simulink model "MIL4L3_SW6_V1_20220211"  (R2018b)
settings: Solver=FixedStepAuto  StartTime=0.0  StopTime=inf  FixedStep=0.001  RelTol=1e-3
PreLoadFcn:
  | A0_MILtest;
undefined symbols (not defined in the file or in its folder): Clb_ICADirect_LaneDisp_StateFive, Clb_ICADirect_LaneDisp_StateFour, Clb_ICADirect_LaneDisp_StateOne, Clb_ICADirect_LaneDisp_StateThree, Clb_ICADirect_LaneDisp_StateTwo, Clb_ICADirect_LaneDisp_StateZero, Clb_ICADirect_LaneDispSW, Clb_ICADirect_TrnLghtsCom_Switch, Clb_ICADirect_TrnLghtsCom_Value, Clb_ICADirect_TrnLghtsCrtl_Inhb, IMAP_Clb_ACU_Driver_Belt, IMAP_Clb_ACU_Driver_Belt_Over, IMAP_Clb_ACU_Passenger_Belt, IMAP_Clb_ACU_Passenger_Belt_Over, IMAP_Clb_ACU_RearLeft_Belt, IMAP_Clb_ACU_RearLeft_Belt_Over, IMAP_Clb_ACU_RearMiddle_Belt, IMAP_Clb_ACU_RearMiddle_Belt_Over, IMAP_Clb_ACU_RearRight_Belt, IMAP_Clb_ACU_RearRight_Belt_Over, IMAP_Clb_AEB_Switch, IMAP_Clb_AEB_Switch_Over, IMAP_Clb_ALC_TLC_Mode, IMAP_Clb_ALC_TLC_Mode_Over, IMAP_Clb_BCM_Battery_Voltage, IMAP_Clb_BCM_Battery_Voltage_Over, IMAP_Clb_BCM_BrakeLamp_State, IMAP_Clb_BCM_BrakeLamp_State_Over, IMAP_Clb_BCM_CHMSL_Status, IMAP_Clb_BCM_CHMSL_Status_Over, IMAP_Clb_BCM_Door_Lock_State, IMAP_Clb_BCM_Door_Lock_State_Over, IMAP_Clb_BCM_FrontWiper_State, IMAP_Clb_BCM_FrontWiper_State_Over, IMAP_Clb_BCM_FrontWiper_Switch, IMAP_Clb_BCM_FrontWiper_Switch_Over, IMAP_Clb_BCM_HazardLamp, IMAP_Clb_BCM_HazardLamp_Over, IMAP_Clb_BCM_HazardLamp_Switch, IMAP_Clb_BCM_HazardLamp_Switch_Over, IMAP_Clb_BCM_HighBeam_State, IMAP_Clb_BCM_HighBeam_State_Over, IMAP_Clb_BCM_Ignition_State, IMAP_Clb_BCM_Ignition_State_Over, IMAP_Clb_BCM_IHBC_Enabled, IMAP_Clb_BCM_IHBC_Enabled_Over, IMAP_Clb_BCM_Left_Light, IMAP_Clb_BCM_Left_Light_Over, IMAP_Clb_BCM_LeftTurn_Switch, IMAP_Clb_BCM_LeftTurn_Switch_Over, IMAP_Clb_BCM_LF_Door_State, IMAP_Clb_BCM_LF_Door_State_Over, IMAP_Clb_BCM_LowBeam_State, IMAP_Clb_BCM_LowBeam_State_Over, IMAP_Clb_BCM_LR_Door_State, IMAP_Clb_BCM_LR_Door_State_Over, IMAP_Clb_BCM_RF_Door_State, IMAP_Clb_BCM_RF_Door_State_Over, IMAP_Clb_BCM_Right_Light, IMAP_Clb_BCM_Right_Light_Over ... (+547)
libraries: CarMaker4SL x2153, simulink x292, dspstat3 x3, canmsglib x2, simulink_extras x1
(part 36 of 52)

== system MIL4L3_SW6_V1_20220211/CarMaker/VehicleControl/OMAP/OMAP1/Runnable_OMAP_10ms_sys/OMAP_Module/ESAS_Direct ==
  note: ESA为扭矩接口。那对应的角度接口的4个信号怎么发？
  Input_ESAS : Inport
  Input_FDMM : Inport  Port=2
  Bus Creator : BusCreator  Inputs=7
  Bus Creator14 : BusCreator  Inputs=8
  Bus Creator23 : BusCreator  Inputs=36
  Bus Creator5 : BusCreator  Inputs=13
  Bus Selector : BusSelector  OutputSignals=ESASve_g_EPS_Factor_Control_convert,ESASve_g_ESA_SWA_CMD_convert,ESASve_y_LKAActivation_convert,ESASve_y_ESA_State_convert,ESASve_y_ESATorqueReq_convert,ESASve_y_ESARequest_convert
  Bus Selector1 : BusSelector  OutputSignals=ESASve_y_ESA_FaultSt_convert
  Constant1 : Constant  Value=0  OutDataTypeStr=uint8
  Constant23 : Constant  Value=0  OutDataTypeStr=uint8
  Constant4 : Constant  Value=0  OutDataTypeStr=uint8
  Data Type Conversion{1..2,4,31} (4 alike) : DataTypeConversion  OutDataTypeStr=uint8
  Data Type Conversion29 : DataTypeConversion  OutDataTypeStr=single
  Data Type Conversion3 : DataTypeConversion  OutDataTypeStr=single
  Data Type Conversion30 : DataTypeConversion  OutDataTypeStr=single
  OMAPve_g_ACCTqReqNum : Constant  Value=-4000  OutDataTypeStr=single
  OMAPve_g_Deceleration_setpoint_deviceNum : Constant  Value=2.05  OutDataTypeStr=single
  OMAPve_g_PotACCTqReqNum : Constant  Value=-4000  OutDataTypeStr=single
  OMAPve_g_TminUp_or_downGearNum : Constant  Value=6.2  OutDataTypeStr=single
  OMAPve_y_ACC_DesiredHeadway_DisplayNum5 : Constant  Value=0  OutDataTypeStr=uint8
  OMAPve_y_ACC_DesiredHeadway_Icon_BasicNum5 : Constant  Value=0  OutDataTypeStr=uint8
  OMAPve_y_ACC_Desired_Set_SpeedNum5 : Constant  Value=0  OutDataTypeStr=uint8
  OMAPve_y_ACC_Engine_Start_RequestNum : Constant  Value=0  OutDataTypeStr=uint8
  OMAPve_y_ACC_HMI_TgtDisp_FlagNum5 : Constant  Value=0  OutDataTypeStr=uint8
  OMAPve_y_ACC_Pop_Up_MessageNum5 : Constant  Value=0  OutDataTypeStr=uint8
  OMAPve_y_ACC_Set_Speed_DisplayNum5 : Constant  Value=0  OutDataTypeStr=uint8
  OMAPve_y_ACC_Vehicle_Icon_DisplayNum5 : Constant  Value=0  OutDataTypeStr=uint8
  OMAPve_y_ADAS_ACCRequestEPBNum : Constant  Value=0  OutDataTypeStr=uint8
  OMAPve_y_ADAS_ELKStsNum1 : Constant  Value=0  OutDataTypeStr=uint8
  OMAPve_y_ADAS_ESCDriveOffNum : Constant  Value=0  OutDataTypeStr=uint8
  OMAPve_y_ADAS_ESCHoldReqNum : Constant  Value=0  OutDataTypeStr=uint8
  OMAPve_y_ADAS_HWAActionSts : Constant  Value=0  OutDataTypeStr=uint8
  OMAPve_y_ADAS_HWAMode : Constant  Value=0  OutDataTypeStr=uint8
  OMAPve_y_ADAS_HWATurnOnIndicator : Constant  Value=0  OutDataTypeStr=uint8
  OMAPve_y_ADAS_ISLCDriverRemind1 : Constant  Value=0  OutDataTypeStr=uint8
  OMAPve_y_ADAS_ISLCState1 : Constant  Value=0  OutDataTypeStr=uint8
  OMAPve_y_ADAS_JAFaultSt_2 : Constant  Value=0  OutDataTypeStr=uint8
  OMAPve_y_ADAS_LightControlValid : Constant  Value=0  OutDataTypeStr=uint8
  OMAPve_y_ADAS_TurnLightsCommand1 : Constant  Value=0  OutDataTypeStr=uint8
  OMAPve_y_AEB_Alert_ReqNum3 : Constant  Value=0  OutDataTypeStr=uint8
  OMAPve_y_AEB_Braking_progressNum : Constant  Value=0  OutDataTypeStr=uint8
  OMAPve_y_AEB_Fault_StatusNum3 : Constant  Value=0  OutDataTypeStr=uint8
  OMAPve_y_AEB_StatusNum : Constant  Value=0  OutDataTypeStr=uint8
  OMAPve_y_AEB_Switch_StatusNum3 : Constant  Value=0  OutDataTypeStr=uint8
  OMAPve_y_AEB_tipsNum3 : Constant  Value=0  OutDataTypeStr=uint8
  OMAPve_y_Decel_RequestNum : Constant  Value=0  OutDataTypeStr=uint8
  OMAPve_y_FCW_StatusNum : Constant  Value=10  OutDataTypeStr=uint8
  OMAPve_y_Function_Acc_statusNum : Constant  Value=3  OutDataTypeStr=uint8
  OMAPve_y_HMI_Popup_StatusNum3 : Constant  Value=0  OutDataTypeStr=uint8
  OMAPve_y_Hands_off_warningNum3 : Constant  Value=0  OutDataTypeStr=uint8
  OMAPve_y_Haptic_AlarmNum : Constant  Value=0  OutDataTypeStr=uint8
  OMAPve_y_ICA_HMI_Txt_DispNum5 : Constant  Value=0  OutDataTypeStr=uint8
  OMAPve_y_LDW_FlagNum4 : Constant  Value=0  OutDataTypeStr=uint8
  OMAPve_y_LDW_Status_DisplayNum4 : Constant  Value=0  OutDataTypeStr=uint8
  OMAPve_y_LKA_Mode_from_CameraNum4 : Constant  Value=0  OutDataTypeStr=uint8
  OMAPve_y_LKA_Status_DisplayNum3 : Constant  Value=0  OutDataTypeStr=uint8
  OMAPve_y_LKA_Switch_StateNum4 : Constant  Value=0  OutDataTypeStr=uint8
  OMAPve_y_LKA_action_indicationNum3 : Constant  Value=0  OutDataTypeStr=uint8
  OMAPve_y_MDD_Decelerationcontrol_requestNum : Constant  Value=0  OutDataTypeStr=uint8
  OMAPve_y_MDD_deceleration_typeNum : Constant  Value=0  OutDataTypeStr=uint8
  OMAPve_y_Powertrain_torquewheel_requestNum : Constant  Value=0  OutDataTypeStr=uint8
  OMAPve_y_Prefill_requestNum : Constant  Value=0  OutDataTypeStr=uint8
  OMAPve_y_RVVACC_Vehiclespeed_request_typeNum5 : Constant  Value=0  OutDataTypeStr=uint8
  OMAPve_y_State_of_the_functionFARC_detNum : Constant  Value=0  OutDataTypeStr=uint8
  OMAPve_y_TARGET_POSITIONNum5 : Constant  Value=6  OutDataTypeStr=uint8
  OMAPve_y_TJA_status_iconNum5 : Constant  Value=0  OutDataTypeStr=uint8
  OMAPve_y_TSR_Vision_Only_Sign_TypeNum5 : Constant  Value=0  OutDataTypeStr=uint8
  OMAPve_y_Vehicle_Lane_DisplayNum4 : Constant  Value=0  OutDataTypeStr=uint8
  OMAPve_y_stAcvTqWhlPTPotReqNum : Constant  Value=0  OutDataTypeStr=uint8
  Terminator1 : Terminator
  ESA_EMS : Outport
  ESA_ESC : Outport  Port=2
  ESA_EPS : Outport  Port=3
  ESA_IC : Outport  Port=4
  wires:
  Bus Creator23/1 -> ESA_IC/1  "ESA_IC"
  Bus Creator14/1 -> ESA_EPS/1  "ESA_EPS"
  OMAPve_y_AEB_Fault_StatusNum3/1 -> Bus Creator23/17  "OMAPve_y_AEB_Fault_Status_2"
  OMAPve_y_ACC_Vehicle_Icon_DisplayNum5/1 -> Bus Creator23/13  "OMAPve_y_ACC_Vehicle_Icon_Display_2"
  OMAPve_y_TSR_Vision_Only_Sign_TypeNum5/1 -> Bus Creator23/8  "OMAPve_y_TSR_Vision_Only_Sign_Type_2"
  OMAPve_y_AEB_Alert_ReqNum3/1 -> Bus Creator23/16  "OMAPve_y_AEB_Alert_Req_2"
  OMAPve_y_TJA_status_iconNum5/1 -> Bus Creator23/36  "OMAPve_y_TJA_status_icon_2"
  OMAPve_y_TARGET_POSITIONNum5/1 -> Bus Creator23/22  "OMAPve_y_TARGET_POSITION_2"
  OMAPve_y_AEB_Switch_StatusNum3/1 -> Bus Creator23/18  "OMAPve_y_AEB_Switch_Status_2"
  OMAPve_y_AEB_tipsNum3/1 -> Bus Creator23/19  "OMAPve_y_AEB_tips_2"
  OMAPve_y_ICA_HMI_Txt_DispNum5/1 -> Bus Creator23/35  "OMAPve_y_ICA_HMI_Txt_Disp_2"
  OMAPve_y_ACC_Desired_Set_SpeedNum5/1 -> Bus Creator23/11  "OMAPve_y_ACC_Desired_Set_Speed_2"
  OMAPve_y_ACC_DesiredHeadway_DisplayNum5/1 -> Bus Creator23/9  "OMAPve_y_ACC_DesiredHeadway_Display_2"
  OMAPve_y_LKA_Switch_StateNum4/1 -> Bus Creator23/32  "OMAPve_y_LKA_Switch_State_2"
  OMAPve_y_LKA_Status_DisplayNum3/1 -> Bus Creator23/31  "OMAPve_y_LKA_Status_Display_2"
  OMAPve_y_LDW_Status_DisplayNum4/1 -> Bus Creator23/29  "OMAPve_y_LDW_Status_Display_2"
  OMAPve_y_ACC_Pop_Up_MessageNum5/1 -> Bus Creator23/15  "OMAPve_y_ACC_Pop_Up_Message_2"
  OMAPve_y_ACC_Set_Speed_DisplayNum5/1 -> Bus Creator23/12  "OMAPve_y_ACC_Set_Speed_Display_2"
  Data Type Conversion30/1 -> Bus Creator14/4  "OMAPve_g_Column_angle_setpoint3F2_2"
  OMAPve_y_HMI_Popup_StatusNum3/1 -> Bus Creator23/26  "OMAPve_y_HMI_Popup_Status_2"
  OMAPve_y_Vehicle_Lane_DisplayNum4/1 -> Bus Creator23/27  "OMAPve_y_Vehicle_Lane_Display_2"
  OMAPve_y_ACC_HMI_TgtDisp_FlagNum5/1 -> Bus Creator23/21  "OMAPve_y_ACC_HMI_TgtDisp_Flag_2"
  Data Type Conversion29/1 -> Bus Creator14/3  "OMAPve_g_Coefficient_toregulate_EPS_2"
  OMAPve_y_Hands_off_warningNum3/1 -> Bus Creator23/25  "OMAPve_y_Hands_off_warning_2"
  OMAPve_y_LKA_action_indicationNum3/1 -> Bus Creator23/33  "OMAPve_y_LKA_action_indication_2"
  OMAPve_y_LKA_Mode_from_CameraNum4/1 -> Bus Creator23/30  "OMAPve_y_LKA_Mode_from_Camera_2"
  Constant1/1 -> Bus Creator14/2  "OMAPve_y_General_state_of_LKA_function3F2_2"
  OMAPve_y_RVVACC_Vehiclespeed_request_typeNum5/1 -> Bus Creator23/14  "OMAPve_y_RVVACC_Vehiclespeed_request_type_2"
  Data Type Conversion31/1 -> Bus Creator14/5  "OMAPve_y_Permit_to_know_if_LKA_or_LPA3F2_2"
  OMAPve_y_LDW_FlagNum4/1 -> Bus Creator23/28  "OMAPve_y_LDW_Flag_2"
  Constant23/1 -> Bus Creator14/1  "OMAPve_y_Power_steering_power_cut3F2_2"
  OMAPve_y_ACC_DesiredHeadway_Icon_BasicNum5/1 -> Bus Creator23/10  "OMAPve_y_ACC_DesiredHeadway_Icon_Basic_2"
  OMAPve_y_State_of_the_functionFARC_detNum/1 -> Bus Creator5/2  "OMAPve_y_State_of_the_functionFARC_det_1"
  OMAPve_y_Haptic_AlarmNum/1 -> Bus Creator5/5  "OMAPve_y_Haptic_Alarm_1"
  OMAPve_y_FCW_StatusNum/1 -> Bus Creator5/1  "OMAPve_y_FCW_Status_1"
  OMAPve_y_MDD_deceleration_typeNum/1 -> Bus Creator5/10  "OMAPve_y_MDD_deceleration_type_1"
  Bus Creator5/1 -> ESA_ESC/1  "ESA_ESC"
  OMAPve_y_MDD_Decelerationcontrol_requestNum/1 -> Bus Creator5/9  "OMAPve_y_MDD_Decelerationcontrol_request_1"
  OMAPve_y_AEB_Braking_progressNum/1 -> Bus Creator5/12  "OMAPve_y_AEB_Braking_progress_1"
  OMAPve_y_AEB_StatusNum/1 -> Bus Creator5/3  "OMAPve_y_AEB_Status_1"
  OMAPve_g_Deceleration_setpoint_deviceNum/1 -> Bus Creator5/8  "OMAPve_g_Deceleration_setpoint_device_1"
  OMAPve_g_ACCTqReqNum/1 -> Bus Creator/3  "OMAPve_g_ACCTqReq_1"
  Bus Creator/1 -> ESA_EMS/1  "ESA_EMS"
  OMAPve_g_PotACCTqReqNum/1 -> Bus Creator/2  "OMAPve_g_PotACCTqReq_1"
  OMAPve_y_ACC_Engine_Start_RequestNum/1 -> Bus Creator/1  "OMAPve_y_ACC_Engine_Start_Request_1"
  OMAPve_y_stAcvTqWhlPTPotReqNum/1 -> Bus Creator/6  "OMAPve_y_stAcvTqWhlPTPotReq_1"
  OMAPve_y_Decel_RequestNum/1 -> Bus Creator5/11  "OMAPve_y_Decel_Request_1"
  OMAPve_y_Function_Acc_statusNum/1 -> Bus Creator/7  "OMAPve_y_Function_Acc_status_1"
  OMAPve_g_TminUp_or_downGearNum/1 -> Bus Creator/5  "OMAPve_g_TminUp_or_downGear_1"
  OMAPve_y_Prefill_requestNum/1 -> Bus Creator5/4  "OMAPve_y_Prefill_request_1"
  OMAPve_y_Powertrain_torquewheel_requestNum/1 -> Bus Creator/4  "OMAPve_y_Powertrain_torquewheel_request_1"
  Input_FDMM/1 -> Terminator1/1
  OMAPve_y_ADAS_ELKStsNum1/1 -> Bus Creator23/34  "OMAPve_y_ADAS_ELKSts_2"
  OMAPve_y_ADAS_ESCHoldReqNum/1 -> Bus Creator5/7  "OMAPve_y_ADAS_ESCHoldReq"
  OMAPve_y_ADAS_ESCDriveOffNum/1 -> Bus Creator5/6  "OMAPve_y_ADAS_ESCDriveOff"
  OMAPve_y_ADAS_ACCRequestEPBNum/1 -> Bus Creator5/13  "OMAPve_y_ADAS_ACCRequestEPB"
  OMAPve_y_ADAS_JAFaultSt_2/1 -> Bus Creator23/20  "OMAPve_y_ADAS_JAFaultSt_2"
  OMAPve_y_ADAS_ISLCState1/1 -> Bus Creator23/23  "OMAPve_y_ADAS_ISLCState_2"
  OMAPve_y_ADAS_ISLCDriverRemind1/1 -> Bus Creator23/24  "OMAPve_y_ADAS_ISLCDriverRemind_2"
  OMAPve_y_ADAS_HWAActionSts/1 -> Bus Creator23/4  "OMAPve_y_ADAS_HWAActionSts_2"
  OMAPve_y_ADAS_HWAMode/1 -> Bus Creator23/7  "OMAPve_y_ADAS_HWAMode_2"
  OMAPve_y_ADAS_TurnLightsCommand1/1 -> Bus Creator23/5  "OMAPve_y_ADAS_TurnLightsCommand_2"
  OMAPve_y_ADAS_HWATurnOnIndicator/1 -> Bus Creator23/3  "OMAPve_y_ADAS_HWATurnOnIndicator_2"
  OMAPve_y_ADAS_LightControlValid/1 -> Bus Creator23/6  "OMAPve_y_ADAS_LightControlValid_2"
  Input_ESAS/1 -> Bus Selector1/1, Bus Selector/1
  Bus Selector/1 -> Data Type Conversion29/1  "<ESASve_g_EPS_Factor_Control_convert>"
  Bus Selector/2 -> Data Type Conversion30/1  "<ESASve_g_ESA_SWA_CMD_convert>"
  Bus Selector/3 -> Data Type Conversion31/1  "<ESASve_y_LKAActivation_convert>"
  Bus Selector/4 -> Data Type Conversion1/1  "<ESASve_y_ESA_State_convert>"
  Data Type Conversion1/1 -> Bus Creator14/6  "OMAPve_y_ADAS_ESAState_2"
  Bus Selector/6 -> Data Type Conversion2/1  "<ESASve_y_ESARequest_convert>"
  Data Type Conversion2/1 -> Bus Creator14/8  "OMAPve_y_ADAS_ESARequest_2"
  Bus Selector/5 -> Data Type Conversion3/1  "<ESASve_y_ESATorqueReq_convert>"
  Data Type Conversion3/1 -> Bus Creator14/7  "OMAPve_g_ADAS_ESATorqueReq_2"
  Data Type Conversion4/1 -> Bus Creator23/2  "OMAPve_y_ADAS_ESAFaultSt_2"
  Bus Selector1/1 -> Data Type Conversion4/1  "<ESASve_y_ESA_FaultSt_convert>"
  Constant4/1 -> Bus Creator23/1  "OMAPve_y_ADAS_ELKPopupMessage_2"

== system MIL4L3_SW6_V1_20220211/CarMaker/VehicleControl/OMAP/OMAP1/Runnable_OMAP_10ms_sys/OMAP_Module/ICA_Direct_G59 ==
  note: 配OMAP_G59
  note: 修改内容：G59 ET0车上与EPS的握手信号
      | 24 :增加转向灯命令信号，并为此信号增加两个标定量
      | 25:首次适配G59HMI，将车道线显示、文字显示、图标显示、声音提示均进行了适配修改，同时新增变道功能相关输出信号OMAPve_y_ADAS_HWATurnOnIndicator_2（请驾驶员拨转向杆确认变道）、OMAPve_y_ADAS_HWAActionSts_2（显示正在往左或是往右变道画面）、OMAPve_y_ADAS_LightControlValid_2（ADAS控转向灯有效性）、OMAPve_y_ADAS_TurnLightsCommand_2（ADAS控转向灯信号）、OMAPve_y_ADAS_HWAMode_2（多车道模式图标信号）。
      | 参考文档：OMAP接口文档3.6、HMI显示需求1.4、信号矩阵V2.1
      | 匹配模型：OMAP_ver032
      | 26:LKA activation控车与否都输出0
      | 27：取消降级达到恢复超时后橙色闪烁的设计，接入ICA模式开关信号、变道打转向灯信号，为HWATurnOnIndicator接入内容
      | 28：驾驶员立即接管触发条件新增车辆非静止
      | 29：经与G35商议一致，取消进入降级时的警示音（handsoffwarning）；把运算中的TH_MODE换为TH_STATE；增加标定量Clb_ICADirect_TrnLghtsCrtl_Inhb指示是否禁止控转向灯
      | 30:当ACC切ICA时，亮黄灯；从头开始开启ICA时，保持亮灰灯
      | 31：把上次改过的ICA icon这一块做了标定量，方便以后调试
      | 32:根据实车测试结果，实施ICA_ICON的更改，优化ACC切ICA时的HMI连续性; 根据对G35等竞品调研，增加扭矩系数变化率相关标定量
      | 33：修改车道线显示模块，显示方式设置两种，简单的只显示双灰双蓝，或者可显示单侧车道线，调试后确定一种；增加显示数值标定量。
      | 34：适配ICAB SW6的输出接口变动，删除部分无用信号，新增变道失败标志位
  Input_ICA : Inport
  Input_FDMM : Inport  Port=2
  Input_IMAP : Inport  Port=3
  ACC_to_ICA : Inport  Port=4
  Bus Creator : BusCreator  Inputs=2
  Bus Creator15 : BusCreator  Inputs=8
  Bus Creator24 : BusCreator  Inputs=36
  Bus Selector : BusSelector  OutputSignals=OMAPve_y_General_state_of_LKA_function3F2_2,OMAPve_g_Coefficient_toregulate_EPS_2,ICABve_g_SteerAngleCmd_convert,OMAPve_y_Permit_to_know_if_LKA_or_LPA3F2_2,ICABve_d_LKATorqueReq_convert,ICABve_g_LKATorqueReq_Value_convert
  Bus Selector1 : BusSelector  OutputSignals=OMAPve_y_ADAS_HWATurnOnIndicator_2,OMAPve_y_ADAS_HWAActionSts_2,OMAPve_y_ADAS_TurnLightsCommand_2,OMAPve_y_ADAS_LightControlValid_2,OMAPve_y_ADAS_HWAMode_2,OMAPve_y_TSR_Vision_Only_Sign_Type_2,OMAPve_y_ISA_Value_2,OMAPve_y_Hands_off_warning_2,OMAPve_y_Vehicle_Lane_Display_2,OMAPve_y_ICA_HMI_Txt_Disp_2,OMAPve_y_TJA_status_icon_2
  Bus Selector2 : BusSelector  OutputSignals=OMAPve_y_ACC_DesiredHeadway_Display_2,OMAPve_y_ACC_DesiredHeadway_Icon_Basic_2,OMAPve_y_ACC_Desired_Set_Speed_2,OMAPve_y_ACC_Set_Speed_Display_2,OMAPve_y_ACC_Vehicle_Icon_Display_2,OMAPve_y_RVVACC_Vehiclespeed_request_type_2,ACCSve_d_ACCMessagePrompt_convert,OMAPve_y_ACC_HMI_TgtDisp_Flag_2,OMAPve_y_TARGET_POSITION_2,ACCSve_d_ACC_ISLCState_convert,ACCSve_d_ACC_ISLCDriverRemind_convert
  Constant{,2..4} (4 alike) : Constant  Value=0  OutDataTypeStr=uint8
  Constant1 : Constant  Value=0  OutDataTypeStr=single
  Constant27 : Constant  Value=34  OutDataTypeStr=uint16
  Data Type Conversion1 : DataTypeConversion  OutDataTypeStr=single
  Data Type Conversion{3..5,7..20,22..25,28,46..47} (24 alike) : DataTypeConversion  OutDataTypeStr=uint8
  Data Type Conversion2 : DataTypeConversion  OutDataTypeStr=single
  Data Type Conversion21 : DataTypeConversion  OutDataTypeStr=single
  ICA_Define : Subsystem
  OMAPve_y_ADAS_ELKStsNum1 : Constant  Value=0  OutDataTypeStr=uint8
  OMAPve_y_ADAS_JAFaultSt_2 : Constant  Value=0  OutDataTypeStr=uint8
  OMAPve_y_AEB_Alert_ReqNum4 : Constant  Value=0  OutDataTypeStr=uint8
  OMAPve_y_AEB_Fault_StatusNum4 : Constant  Value=0  OutDataTypeStr=uint8
  OMAPve_y_AEB_Switch_StatusNum4 : Constant  Value=0  OutDataTypeStr=uint8
  OMAPve_y_AEB_tipsNum4 : Constant  Value=0  OutDataTypeStr=uint8
  OMAPve_y_HMI_Popup_StatusNum4 : Constant  Value=0  OutDataTypeStr=uint8
  OMAPve_y_LDW_FlagNum5 : Constant  Value=0  OutDataTypeStr=uint8
  OMAPve_y_LDW_Status_DisplayNum5 : Constant  Value=0  OutDataTypeStr=uint8
  OMAPve_y_LKA_Mode_from_CameraNum5 : Constant  Value=0  OutDataTypeStr=uint8
  OMAPve_y_LKA_Status_DisplayNum4 : Constant  Value=0  OutDataTypeStr=uint8
  OMAPve_y_LKA_Switch_StateNum5 : Constant  Value=0  OutDataTypeStr=uint8
  OMAPve_y_LKA_action_indicationNum4 : Constant  Value=0  OutDataTypeStr=uint8
  OMAPve_y_Power_steering_power_cut3F2Num2 : Constant  Value=0  OutDataTypeStr=uint8
  Terminator : Terminator
  Terminator1 : Terminator
  Terminator2 : Terminator
  ICA_EPS : Outport
  ICA_IC : Outport  Port=2
  ICA_Input : Outport  Port=3
  wires:
  OMAPve_y_AEB_Alert_ReqNum4/1 -> Bus Creator24/16  "OMAPve_y_AEB_Alert_Req_2"
  Data Type Conversion16/1 -> Bus Creator24/14  "OMAPve_y_RVVACC_Vehiclespeed_request_type_2"
  Bus Selector1/8 -> Data Type Conversion7/1  "<OMAPve_y_Hands_off_warning_2>"
  Data Type Conversion12/1 -> Bus Creator24/10  "OMAPve_y_ACC_DesiredHeadway_Icon_Basic_2"
  Bus Selector1/7 -> ?  "<OMAPve_y_ISA_Value_2>"
  Data Type Conversion14/1 -> Bus Creator24/12  "OMAPve_y_ACC_Set_Speed_Display_2"
  OMAPve_y_LDW_FlagNum5/1 -> Bus Creator24/28  "OMAPve_y_LDW_Flag_2"
  Bus Creator24/1 -> ICA_IC/1  "ICA_IC"
  OMAPve_y_AEB_tipsNum4/1 -> Bus Creator24/19  "OMAPve_y_AEB_tips_2"
  Bus Selector1/11 -> Data Type Conversion9/1  "<OMAPve_y_TJA_status_icon_2>"
  Data Type Conversion13/1 -> Bus Creator24/11  "OMAPve_y_ACC_Desired_Set_Speed_2"
  OMAPve_y_LKA_Status_DisplayNum4/1 -> Bus Creator24/31  "OMAPve_y_LKA_Status_Display_2"
  Data Type Conversion18/1 -> Bus Creator24/21  "OMAPve_y_ACC_HMI_TgtDisp_Flag_2"
  Data Type Conversion17/1 -> Bus Creator24/15  "OMAPve_y_ACC_Pop_Up_Message_2"
  OMAPve_y_LKA_Switch_StateNum5/1 -> Bus Creator24/32  "OMAPve_y_LKA_Switch_State_2"
  Data Type Conversion15/1 -> Bus Creator24/13  "OMAPve_y_ACC_Vehicle_Icon_Display_2"
  Bus Selector1/10 -> Data Type Conversion10/1  "<OMAPve_y_ICA_HMI_Txt_Disp_2>"
  OMAPve_y_LKA_Mode_from_CameraNum5/1 -> Bus Creator24/30  "OMAPve_y_LKA_Mode_from_Camera_2"
  OMAPve_y_LDW_Status_DisplayNum5/1 -> Bus Creator24/29  "OMAPve_y_LDW_Status_Display_2"
  OMAPve_y_AEB_Fault_StatusNum4/1 -> Bus Creator24/17  "OMAPve_y_AEB_Fault_Status_2"
  Bus Selector1/6 -> Data Type Conversion4/1  "<OMAPve_y_TSR_Vision_Only_Sign_Type_2>"
  OMAPve_y_HMI_Popup_StatusNum4/1 -> Bus Creator24/26  "OMAPve_y_HMI_Popup_Status_2"
  Bus Creator15/1 -> ICA_EPS/1  "ICA_EPS"
  Data Type Conversion11/1 -> Bus Creator24/9  "OMAPve_y_ACC_DesiredHeadway_Display_2"
  Data Type Conversion19/1 -> Bus Creator24/22  "OMAPve_y_TARGET_POSITION_2"
  OMAPve_y_AEB_Switch_StatusNum4/1 -> Bus Creator24/18  "OMAPve_y_AEB_Switch_Status_2"
  OMAPve_y_LKA_action_indicationNum4/1 -> Bus Creator24/33  "OMAPve_y_LKA_action_indication_2"
  Bus Selector1/9 -> Data Type Conversion8/1  "<OMAPve_y_Vehicle_Lane_Display_2>"
  Input_ICA/1 -> ICA_Define/1(In1)
  Input_IMAP/1 -> ICA_Define/3(In2)
  Input_FDMM/1 -> ICA_Define/2(In3)
  ACC_to_ICA/1 -> Bus Selector2/1, ICA_Define/4(In4)
  ICA_Define/2(Out2) -> Bus Creator/2, Bus Selector1/1  "HMI"
  Bus Creator/1 -> ICA_Input/1
  Data Type Conversion4/1 -> Bus Creator24/8  "OMAPve_y_TSR_Vision_Only_Sign_Type_2"
  Data Type Conversion7/1 -> Bus Creator24/25  "OMAPve_y_Hands_off_warning_2"
  Data Type Conversion8/1 -> Bus Creator24/27  "OMAPve_y_Vehicle_Lane_Display_2"
  Data Type Conversion9/1 -> Bus Creator24/36  "OMAPve_y_TJA_status_icon_2"
  Data Type Conversion10/1 -> Bus Creator24/35  "OMAPve_y_ICA_HMI_Txt_Disp_2"
  Bus Selector2/1 -> Data Type Conversion11/1  "<OMAPve_y_ACC_DesiredHeadway_Display_2>"
  Bus Selector2/2 -> Data Type Conversion12/1  "<OMAPve_y_ACC_DesiredHeadway_Icon_Basic_2>"
  Bus Selector2/3 -> Data Type Conversion13/1  "<OMAPve_y_ACC_Desired_Set_Speed_2>"
  Bus Selector2/4 -> Data Type Conversion14/1  "<OMAPve_y_ACC_Set_Speed_Display_2>"
  Bus Selector2/5 -> Data Type Conversion15/1  "<OMAPve_y_ACC_Vehicle_Icon_Display_2>"
  Bus Selector2/6 -> Data Type Conversion16/1  "<OMAPve_y_RVVACC_Vehiclespeed_request_type_2>"
  Bus Selector2/7 -> Data Type Conversion17/1  "<ACCSve_d_ACCMessagePrompt_convert>"
  Bus Selector2/8 -> Data Type Conversion18/1  "<OMAPve_y_ACC_HMI_TgtDisp_Flag_2>"
  Bus Selector2/9 -> Data Type Conversion19/1  "<OMAPve_y_TARGET_POSITION_2>"
  OMAPve_y_ADAS_ELKStsNum1/1 -> Bus Creator24/34  "OMAPve_y_ADAS_ELKSts_2"
  Data Type Conversion3/1 -> Bus Creator15/5  "OMAPve_y_Permit_to_know_if_LKA_or_LPA3F2_2"
  Bus Selector/5 -> Data Type Conversion20/1  "<ICABve_d_LKATorqueReq_convert>"
  Bus Selector/1 -> Data Type Conversion28/1  "<OMAPve_y_General_state_of_LKA_function3F2_2>"
  Bus Selector/4 -> Data Type Conversion3/1  "<OMAPve_y_Permit_to_know_if_LKA_or_LPA3F2_2>"
  Bus Selector/6 -> Data Type Conversion21/1  "<ICABve_g_LKATorqueReq_Value_convert>"
  Data Type Conversion20/1 -> Terminator/1  "OMAPve_y_DAS4_Status_LKATorqueReq"
  Bus Selector/2 -> Data Type Conversion1/1  "<OMAPve_g_Coefficient_toregulate_EPS_2>"
  OMAPve_y_Power_steering_power_cut3F2Num2/1 -> Bus Creator15/1  "OMAPve_y_Power_steering_power_cut3F2_2"
  Data Type Conversion1/1 -> Bus Creator15/3  "OMAPve_g_Coefficient_toregulate_EPS_2"
  Data Type Conversion28/1 -> Bus Creator15/2  "OMAPve_y_General_state_of_LKA_function3F2_2"
  Data Type Conversion21/1 -> Terminator1/1  "OMAPve_g_DAS4_Status_LKATorqueReq_Value"
  ICA_Define/1(Out1) -> Bus Selector/1, Bus Creator/1  "actuator"
  Bus Selector/3 -> Data Type Conversion2/1  "<ICABve_g_SteerAngleCmd_convert>"
  Data Type Conversion2/1 -> Bus Creator15/4  "OMAPve_g_Column_angle_setpoint3F2_2"
  Constant27/1 -> Terminator2/1  "ob_OMAP_ICAdirect_version"
  OMAPve_y_ADAS_JAFaultSt_2/1 -> Bus Creator24/20  "OMAPve_y_ADAS_JAFaultSt_2"
  Bus Selector1/3 -> Data Type Conversion5/1  "<OMAPve_y_ADAS_TurnLightsCommand_2>"
  Data Type Conversion5/1 -> Bus Creator24/5  "OMAPve_y_ADAS_TurnLightsCommand_2"
  Bus Selector1/1 -> Data Type Conversion22/1  "<OMAPve_y_ADAS_HWATurnOnIndicator_2>"
  Data Type Conversion22/1 -> Bus Creator24/3  "OMAPve_y_ADAS_HWATurnOnIndicator_2"
  Data Type Conversion23/1 -> Bus Creator24/4  "OMAPve_y_ADAS_HWAActionSts_2"
  Bus Selector1/2 -> Data Type Conversion23/1  "<OMAPve_y_ADAS_HWAActionSts_2>"
  Data Type Conversion24/1 -> Bus Creator24/6  "OMAPve_y_ADAS_LightControlValid_2"
  Bus Selector1/4 -> Data Type Conversion24/1  "<OMAPve_y_ADAS_LightControlValid_2>"
  Bus Selector1/5 -> Data Type Conversion25/1  "<OMAPve_y_ADAS_HWAMode_2>"
  Data Type Conversion25/1 -> Bus Creator24/7  "OMAPve_y_ADAS_HWAMode_2"
  Data Type Conversion47/1 -> Bus Creator24/24  "OMAPve_y_ADAS_ISLCDriverRemind_2"
  Data Type Conversion46/1 -> Bus Creator24/23  "OMAPve_y_ADAS_ISLCState_2"
  Bus Selector2/10 -> Data Type Conversion46/1  "<ACCSve_d_ACC_ISLCState_convert>"
  Bus Selector2/11 -> Data Type Conversion47/1  "<ACCSve_d_ACC_ISLCDriverRemind_convert>"
  Constant1/1 -> Bus Creator15/7  "OMAPve_g_ADAS_ESATorqueReq_2"
  Constant/1 -> Bus Creator15/6  "OMAPve_y_ADAS_ESAState_2"
  Constant2/1 -> Bus Creator15/8  "OMAPve_y_ADAS_ESARequest_2"
  Constant3/1 -> Bus Creator24/2  "OMAPve_y_ADAS_ESAFaultSt_2"
  Constant4/1 -> Bus Creator24/1  "OMAPve_y_ADAS_ELKPopupMessage_2"

== system MIL4L3_SW6_V1_20220211/CarMaker/VehicleControl/OMAP/OMAP1/Runnable_OMAP_10ms_sys/OMAP_Module/JABS_Direct ==
  Input_JABS : Inport
  Input_FDMM : Inport  Port=2
  Bus Creator10 : BusCreator  Inputs=8
  Bus Creator20 : BusCreator  Inputs=36
  Bus Creator4 : BusCreator  Inputs=7
  Bus Creator9 : BusCreator  Inputs=13
  Bus Selector8 : BusSelector  OutputSignals=JABSve_d_DbJACWStatus_convert,JABSve_d_DbFunFARCSta_convert,JABSve_d_DbPrefillReq_convert,JABSve_d_DbHapticAlarm_convert,JABSve_d_DbESCDriveOff_convert,JABSve_d_DbESCHoldReq_convert,JABSve_g_DbDecSetpoint_convert,JABSve_d_DbMDDdecRequest_convert,JABSve_d_DbMDDdecType_convert,JABSve_d_DbBraking_progress_convert,JABSve_d_DbAlertReq_convert,JABSve_d_DbSwitchStatus_convert,JABSve_d_DbTips_convert,JABSve_d_DbFltStatus_convert
  Constant{,2..4,14,16,19} (7 alike) : Constant  Value=0  OutDataTypeStr=uint8
  Constant1 : Constant  Value=0  OutDataTypeStr=single
  Constant13 : Constant  Value=6.2  OutDataTypeStr=single
  Constant15 : Constant  Value=3  OutDataTypeStr=uint8
  Constant17 : Constant  Value=-4000  OutDataTypeStr=single
  Constant18 : Constant  Value=-4000  OutDataTypeStr=single
  Data Type Conversion{1..3,15..24,26..27} (15 alike) : DataTypeConversion  OutDataTypeStr=uint8
  Data Type Conversion14 : DataTypeConversion  OutDataTypeStr=single
  OMAPve_g_Coefficient_toregulate_EPSNum : Constant  Value=0  OutDataTypeStr=single
  OMAPve_g_Column_angle_setpoint3F2Num : Constant  Value=0  OutDataTypeStr=single
  OMAPve_y_ACC_DesiredHeadway_DisplayNum2 : Constant  Value=0  OutDataTypeStr=uint8
  OMAPve_y_ACC_DesiredHeadway_Icon_BasicNum2 : Constant  Value=0  OutDataTypeStr=uint8
  OMAPve_y_ACC_Desired_Set_SpeedNum2 : Constant  Value=0  OutDataTypeStr=uint8
  OMAPve_y_ACC_HMI_TgtDisp_FlagNum2 : Constant  Value=0  OutDataTypeStr=uint8
  OMAPve_y_ACC_Pop_Up_MessageNum2 : Constant  Value=0  OutDataTypeStr=uint8
  OMAPve_y_ACC_Set_Speed_DisplayNum2 : Constant  Value=0  OutDataTypeStr=uint8
  OMAPve_y_ACC_Vehicle_Icon_DisplayNum2 : Constant  Value=0  OutDataTypeStr=uint8
  OMAPve_y_ADAS_ACCRequestEPBNum : Constant  Value=0  OutDataTypeStr=uint8
  OMAPve_y_ADAS_ELKStsNum1 : Constant  Value=0  OutDataTypeStr=uint8
  OMAPve_y_ADAS_HWAActionSts : Constant  Value=0  OutDataTypeStr=uint8
  OMAPve_y_ADAS_HWAMode : Constant  Value=0  OutDataTypeStr=uint8
  OMAPve_y_ADAS_HWATurnOnIndicator : Constant  Value=0  OutDataTypeStr=uint8
  OMAPve_y_ADAS_ISLCDriverRemind1 : Constant  Value=0  OutDataTypeStr=uint8
  OMAPve_y_ADAS_ISLCState1 : Constant  Value=0  OutDataTypeStr=uint8
  OMAPve_y_ADAS_LightControlValid : Constant  Value=0  OutDataTypeStr=uint8
  OMAPve_y_ADAS_TurnLightsCommand2 : Constant  Value=0  OutDataTypeStr=uint8
  OMAPve_y_AEB_Fault_Status_2 : Constant  Value=0  OutDataTypeStr=uint8
  OMAPve_y_General_state_of_LKA_function3F2Num : Constant  Value=0  OutDataTypeStr=uint8
  OMAPve_y_HMI_Popup_StatusNum2 : Constant  Value=0  OutDataTypeStr=uint8
  OMAPve_y_Hands_off_warningNum2 : Constant  Value=0  OutDataTypeStr=uint8
  OMAPve_y_ICA_HMI_Txt_DispNum2 : Constant  Value=0  OutDataTypeStr=uint8
  OMAPve_y_LDW_FlagNum2 : Constant  Value=0  OutDataTypeStr=uint8
  OMAPve_y_LDW_Status_DisplayNum2 : Constant  Value=0  OutDataTypeStr=uint8
  OMAPve_y_LKA_Mode_from_CameraNum2 : Constant  Value=0  OutDataTypeStr=uint8
  OMAPve_y_LKA_Status_DisplayNum2 : Constant  Value=0  OutDataTypeStr=uint8
  OMAPve_y_LKA_Switch_StateNum2 : Constant  Value=0  OutDataTypeStr=uint8
  OMAPve_y_LKA_action_indicationNum2 : Constant  Value=0  OutDataTypeStr=uint8
  OMAPve_y_Permit_to_know_if_LKA_or_LPA3F2Num : Constant  Value=0  OutDataTypeStr=uint8
  OMAPve_y_Power_steering_power_cut3F2Num : Constant  Value=0  OutDataTypeStr=uint8
  OMAPve_y_RVVACC_Vehiclespeed_request_typeNum2 : Constant  Value=0  OutDataTypeStr=uint8
  OMAPve_y_TARGET_POSITIONNum2 : Constant  Value=6  OutDataTypeStr=uint8
  OMAPve_y_TJA_status_iconNum2 : Constant  Value=0  OutDataTypeStr=uint8
  OMAPve_y_TSR_Vision_Only_Sign_TypeNum2 : Constant  Value=0  OutDataTypeStr=uint8
  OMAPve_y_Vehicle_Lane_DisplayNum2 : Constant  Value=0  OutDataTypeStr=uint8
  Terminator : Terminator
  JA_EMS : Outport
  JA_ESC : Outport  Port=2
  JA_EPS : Outport  Port=3
  JA_IC : Outport  Port=4
  JA_Input : Outport  Port=5
  wires:
  Bus Creator20/1 -> JA_IC/1  "JA_IC"
  Bus Selector8/12 -> Data Type Conversion26/1  "<JABSve_d_DbSwitchStatus_convert>"
  Bus Selector8/13 -> Data Type Conversion27/1  "<JABSve_d_DbTips_convert>"
  Bus Selector8/9 -> Data Type Conversion17/1  "<JABSve_d_DbMDDdecType_convert>"
  Data Type Conversion27/1 -> Bus Creator20/19  "OMAPve_y_AEB_tips_2"
  OMAPve_y_ICA_HMI_Txt_DispNum2/1 -> Bus Creator20/35  "OMAPve_y_ICA_HMI_Txt_Disp_2"
  OMAPve_y_TARGET_POSITIONNum2/1 -> Bus Creator20/22  "OMAPve_y_TARGET_POSITION_2"
  OMAPve_y_ACC_Vehicle_Icon_DisplayNum2/1 -> Bus Creator20/13  "OMAPve_y_ACC_Vehicle_Icon_Display_2"
  Bus Selector8/4 -> Data Type Conversion23/1  "<JABSve_d_DbHapticAlarm_convert>"
  OMAPve_y_HMI_Popup_StatusNum2/1 -> Bus Creator20/26  "OMAPve_y_HMI_Popup_Status_2"
  OMAPve_y_LKA_Status_DisplayNum2/1 -> Bus Creator20/31  "OMAPve_y_LKA_Status_Display_2"
  OMAPve_y_ACC_DesiredHeadway_DisplayNum2/1 -> Bus Creator20/9  "OMAPve_y_ACC_DesiredHeadway_Display_2"
  OMAPve_y_AEB_Fault_Status_2/1 -> Bus Creator20/17  "OMAPve_y_AEB_Fault_Status_2"
  Data Type Conversion24/1 -> Bus Creator20/16  "OMAPve_y_AEB_Alert_Req_2"
  OMAPve_y_ACC_HMI_TgtDisp_FlagNum2/1 -> Bus Creator20/21  "OMAPve_y_ACC_HMI_TgtDisp_Flag_2"
  Input_JABS/1 -> JA_Input/1, Bus Selector8/1
  OMAPve_y_LKA_Mode_from_CameraNum2/1 -> Bus Creator20/30  "OMAPve_y_LKA_Mode_from_Camera_2"
  Bus Selector8/11 -> Data Type Conversion24/1  "<JABSve_d_DbAlertReq_convert>"
  OMAPve_y_Vehicle_Lane_DisplayNum2/1 -> Bus Creator20/27  "OMAPve_y_Vehicle_Lane_Display_2"
  OMAPve_y_LKA_action_indicationNum2/1 -> Bus Creator20/33  "OMAPve_y_LKA_action_indication_2"
  Bus Selector8/1 -> Data Type Conversion22/1  "<JABSve_d_DbJACWStatus_convert>"
  Data Type Conversion15/1 -> Bus Creator9/9  "OMAPve_y_MDD_Decelerationcontrol_request_1"
  OMAPve_y_ACC_Desired_Set_SpeedNum2/1 -> Bus Creator20/11  "OMAPve_y_ACC_Desired_Set_Speed_2"
  OMAPve_y_TSR_Vision_Only_Sign_TypeNum2/1 -> Bus Creator20/8  "OMAPve_y_TSR_Vision_Only_Sign_Type_2"
  Constant15/1 -> Bus Creator4/7  "OMAPve_y_Function_Acc_status_1"
  Bus Creator4/1 -> JA_EMS/1  "JA_EMS"
  Constant13/1 -> Bus Creator4/5  "OMAPve_g_TminUp_or_downGear_1"
  OMAPve_y_LDW_Status_DisplayNum2/1 -> Bus Creator20/29  "OMAPve_y_LDW_Status_Display_2"
  Data Type Conversion26/1 -> Bus Creator20/18  "OMAPve_y_AEB_Switch_Status_2"
  Data Type Conversion22/1 -> Bus Creator9/1  "OMAPve_y_FCW_Status_1"
  Data Type Conversion17/1 -> Bus Creator9/10  "OMAPve_y_MDD_deceleration_type_1"
  Data Type Conversion14/1 -> Bus Creator9/8  "OMAPve_g_Deceleration_setpoint_device_1"
  Bus Selector8/3 -> Data Type Conversion16/1  "<JABSve_d_DbPrefillReq_convert>"
  Constant14/1 -> Bus Creator4/6  "OMAPve_y_stAcvTqWhlPTPotReq_1"
  Bus Selector8/8 -> Data Type Conversion20/1, Data Type Conversion15/1, Data Type Conversion21/1  "<JABSve_d_DbMDDdecRequest_convert>"
  Bus Creator9/1 -> JA_ESC/1  "JA_ESC"
  Constant16/1 -> Bus Creator4/1  "OMAPve_y_ACC_Engine_Start_Request_1"
  OMAPve_y_LKA_Switch_StateNum2/1 -> Bus Creator20/32  "OMAPve_y_LKA_Switch_State_2"
  OMAPve_y_ACC_DesiredHeadway_Icon_BasicNum2/1 -> Bus Creator20/10  "OMAPve_y_ACC_DesiredHeadway_Icon_Basic_2"
  OMAPve_y_LDW_FlagNum2/1 -> Bus Creator20/28  "OMAPve_y_LDW_Flag_2"
  Data Type Conversion16/1 -> Bus Creator9/4  "OMAPve_y_Prefill_request_1"
  Data Type Conversion18/1 -> Bus Creator9/2  "OMAPve_y_State_of_the_functionFARC_det_1"
  Constant19/1 -> Bus Creator4/4  "OMAPve_y_Powertrain_torquewheel_request_1"
  Data Type Conversion23/1 -> Bus Creator9/5  "OMAPve_y_Haptic_Alarm_1"
  Data Type Conversion19/1 -> Bus Creator9/3  "OMAPve_y_AEB_Status_1"
  OMAPve_y_RVVACC_Vehiclespeed_request_typeNum2/1 -> Bus Creator20/14  "OMAPve_y_RVVACC_Vehiclespeed_request_type_2"
  Bus Selector8/7 -> Data Type Conversion14/1  "<JABSve_g_DbDecSetpoint_convert>"
  Constant18/1 -> Bus Creator4/3  "OMAPve_g_ACCTqReq_1"
  OMAPve_y_Hands_off_warningNum2/1 -> Bus Creator20/25  "OMAPve_y_Hands_off_warning_2"
  OMAPve_y_TJA_status_iconNum2/1 -> Bus Creator20/36  "OMAPve_y_TJA_status_icon_2"
  Constant17/1 -> Bus Creator4/2  "OMAPve_g_PotACCTqReq_1"
  OMAPve_y_ACC_Pop_Up_MessageNum2/1 -> Bus Creator20/15  "OMAPve_y_ACC_Pop_Up_Message_2"
  Bus Selector8/2 -> Data Type Conversion19/1, Data Type Conversion18/1  "<JABSve_d_DbFunFARCSta_convert>"
  Data Type Conversion20/1 -> Bus Creator9/11  "OMAPve_y_Decel_Request_1"
  OMAPve_y_ACC_Set_Speed_DisplayNum2/1 -> Bus Creator20/12  "OMAPve_y_ACC_Set_Speed_Display_2"
  Data Type Conversion21/1 -> Bus Creator9/12  "OMAPve_y_AEB_Braking_progress_1"
  OMAPve_y_Power_steering_power_cut3F2Num/1 -> Bus Creator10/1  "OMAPve_y_Power_steering_power_cut3F2_2"
  Bus Creator10/1 -> JA_EPS/1  "JA_EPS"
  OMAPve_y_Permit_to_know_if_LKA_or_LPA3F2Num/1 -> Bus Creator10/5  "OMAPve_y_Permit_to_know_if_LKA_or_LPA3F2_2"
  OMAPve_g_Coefficient_toregulate_EPSNum/1 -> Bus Creator10/3  "OMAPve_g_Coefficient_toregulate_EPS_2"
  OMAPve_y_General_state_of_LKA_function3F2Num/1 -> Bus Creator10/2  "OMAPve_y_General_state_of_LKA_function3F2_2"
  OMAPve_g_Column_angle_setpoint3F2Num/1 -> Bus Creator10/4  "OMAPve_g_Column_angle_setpoint3F2_2"
  Input_FDMM/1 -> Terminator/1
  OMAPve_y_ADAS_ELKStsNum1/1 -> Bus Creator20/34  "OMAPve_y_ADAS_ELKSts_2"
  Data Type Conversion2/1 -> Bus Creator9/7  "OMAPve_y_ADAS_ESCHoldReq"
  Data Type Conversion1/1 -> Bus Creator9/6  "OMAPve_y_ADAS_ESCDriveOff"
  OMAPve_y_ADAS_ACCRequestEPBNum/1 -> Bus Creator9/13  "OMAPve_y_ADAS_ACCRequestEPB"
  Bus Selector8/5 -> Data Type Conversion1/1  "<JABSve_d_DbESCDriveOff_convert>"
  Bus Selector8/6 -> Data Type Conversion2/1  "<JABSve_d_DbESCHoldReq_convert>"
  Bus Selector8/10 -> ?  "<JABSve_d_DbBraking_progress_convert>"
  Data Type Conversion3/1 -> Bus Creator20/20  "OMAPve_y_ADAS_JAFaultSt_2"
  Bus Selector8/14 -> Data Type Conversion3/1  "<JABSve_d_DbFltStatus_convert>"
  OMAPve_y_ADAS_ISLCState1/1 -> Bus Creator20/23  "OMAPve_y_ADAS_ISLCState_2"
  OMAPve_y_ADAS_ISLCDriverRemind1/1 -> Bus Creator20/24  "OMAPve_y_ADAS_ISLCDriverRemind_2"
  OMAPve_y_ADAS_LightControlValid/1 -> Bus Creator20/6  "OMAPve_y_ADAS_LightControlValid_2"
  OMAPve_y_ADAS_HWAActionSts/1 -> Bus Creator20/4  "OMAPve_y_ADAS_HWAActionSts_2"
  OMAPve_y_ADAS_HWATurnOnIndicator/1 -> Bus Creator20/3  "OMAPve_y_ADAS_HWATurnOnIndicator_2"
  OMAPve_y_ADAS_HWAMode/1 -> Bus Creator20/7  "OMAPve_y_ADAS_HWAMode_2"
  OMAPve_y_ADAS_TurnLightsCommand2/1 -> Bus Creator20/5  "OMAPve_y_ADAS_TurnLightsCommand_2"
  Constant1/1 -> Bus Creator10/7  "OMAPve_g_ADAS_ESATorqueReq_2"
  Constant/1 -> Bus Creator10/6  "OMAPve_y_ADAS_ESAState_2"
  Constant2/1 -> Bus Creator10/8  "OMAPve_y_ADAS_ESARequest_2"
  Constant3/1 -> Bus Creator20/2  "OMAPve_y_ADAS_ESAFaultSt_2"
  Constant4/1 -> Bus Creator20/1  "OMAPve_y_ADAS_ELKPopupMessage_2"

== system MIL4L3_SW6_V1_20220211/CarMaker/VehicleControl/OMAP/OMAP1/Runnable_OMAP_10ms_sys/OMAP_Module/LKAS_Direct ==
  Input_LKAS : Inport
  Input_FDMM : Inport  Port=2
  Bus Creator : BusCreator  Inputs=7
  Bus Creator1 : BusCreator  Inputs=36
  Bus Creator12 : BusCreator  Inputs=8
  Bus Creator5 : BusCreator  Inputs=13
  Bus Selector : BusSelector  OutputSignals=FDMMve_d_LkaFcnConf_convert
  Bus Selector9 : BusSelector  OutputSignals=LKASve_y_EPS_State_Control_convert,LKASve_g_EPS_Factor_Control_convert,LKASve_g_LKA_SWA_Control_convert,LKASve_y_EPS_LKA_Control_convert,LKASve_y_Hands_Off_Warning_convert,LKASve_y_HMI_Popup_Status_convert,LKASve_y_Vehicle_Lane_Display_convert,LKASve_y_LDW_Flag_convert,LKASve_y_LDW_Status_Display_convert,LKASve_y_LKA_Status_Display_convert,LKASve_y_LKA_Action_Indication_convert
  Constant{,2..3,5,21..22} (6 alike) : Constant  Value=0  OutDataTypeStr=uint8
  Constant1 : Constant  Value=0  OutDataTypeStr=single
  Data Type Conversion{28,31..39} (10 alike) : DataTypeConversion  OutDataTypeStr=uint8
  Data Type Conversion29 : DataTypeConversion  OutDataTypeStr=single
  Data Type Conversion30 : DataTypeConversion  OutDataTypeStr=single
  OMAPve_g_ACCTqReqNum : Constant  Value=-4000  OutDataTypeStr=single
  OMAPve_g_Deceleration_setpoint_deviceNum : Constant  Value=2.05  OutDataTypeStr=single
  OMAPve_g_PotACCTqReqNum : Constant  Value=-4000  OutDataTypeStr=single
  OMAPve_g_TminUp_or_downGearNum : Constant  Value=6.2  OutDataTypeStr=single
  OMAPve_y_ACC_DesiredHeadway_DisplayNum3 : Constant  Value=0  OutDataTypeStr=uint8
  OMAPve_y_ACC_DesiredHeadway_Icon_BasicNum3 : Constant  Value=0  OutDataTypeStr=uint8
  OMAPve_y_ACC_Desired_Set_SpeedNum3 : Constant  Value=0  OutDataTypeStr=uint8
  OMAPve_y_ACC_Engine_Start_RequestNum : Constant  Value=0  OutDataTypeStr=uint8
  OMAPve_y_ACC_HMI_TgtDisp_FlagNum3 : Constant  Value=0  OutDataTypeStr=uint8
  OMAPve_y_ACC_Pop_Up_MessageNum3 : Constant  Value=0  OutDataTypeStr=uint8
  OMAPve_y_ACC_Set_Speed_DisplayNum3 : Constant  Value=0  OutDataTypeStr=uint8
  OMAPve_y_ACC_Vehicle_Icon_DisplayNum3 : Constant  Value=0  OutDataTypeStr=uint8
  OMAPve_y_ADAS_ACCRequestEPBNum : Constant  Value=0  OutDataTypeStr=uint8
  OMAPve_y_ADAS_ELKStsNum1 : Constant  Value=0  OutDataTypeStr=uint8
  OMAPve_y_ADAS_ESCDriveOffNum : Constant  Value=0  OutDataTypeStr=uint8
  OMAPve_y_ADAS_ESCHoldReqNum : Constant  Value=0  OutDataTypeStr=uint8
  OMAPve_y_ADAS_HWAActionSts : Constant  Value=0  OutDataTypeStr=uint8
  OMAPve_y_ADAS_HWAMode : Constant  Value=0  OutDataTypeStr=uint8
  OMAPve_y_ADAS_HWATurnOnIndicator : Constant  Value=0  OutDataTypeStr=uint8
  OMAPve_y_ADAS_ISLCDriverRemind1 : Constant  Value=0  OutDataTypeStr=uint8
  OMAPve_y_ADAS_ISLCState1 : Constant  Value=0  OutDataTypeStr=uint8
  OMAPve_y_ADAS_JAFaultSt_2 : Constant  Value=0  OutDataTypeStr=uint8
  OMAPve_y_ADAS_LightControlValid : Constant  Value=0  OutDataTypeStr=uint8
  OMAPve_y_ADAS_TurnLightsCommand1 : Constant  Value=0  OutDataTypeStr=uint8
  OMAPve_y_AEB_Alert_ReqNum1 : Constant  Value=0  OutDataTypeStr=uint8
  OMAPve_y_AEB_Braking_progressNum : Constant  Value=0  OutDataTypeStr=uint8
  OMAPve_y_AEB_Fault_StatusNum1 : Constant  Value=0  OutDataTypeStr=uint8
  OMAPve_y_AEB_StatusNum : Constant  Value=0  OutDataTypeStr=uint8
  OMAPve_y_AEB_Switch_StatusNum1 : Constant  Value=0  OutDataTypeStr=uint8
  OMAPve_y_AEB_tipsNum1 : Constant  Value=0  OutDataTypeStr=uint8
  OMAPve_y_Decel_RequestNum : Constant  Value=0  OutDataTypeStr=uint8
  OMAPve_y_FCW_StatusNum : Constant  Value=10  OutDataTypeStr=uint8
  OMAPve_y_Function_Acc_statusNum : Constant  Value=3  OutDataTypeStr=uint8
  OMAPve_y_Haptic_AlarmNum : Constant  Value=0  OutDataTypeStr=uint8
  OMAPve_y_ICA_HMI_Txt_DispNum3 : Constant  Value=0  OutDataTypeStr=uint8
  OMAPve_y_MDD_Decelerationcontrol_requestNum : Constant  Value=0  OutDataTypeStr=uint8
  OMAPve_y_MDD_deceleration_typeNum : Constant  Value=0  OutDataTypeStr=uint8
  OMAPve_y_Powertrain_torquewheel_requestNum : Constant  Value=0  OutDataTypeStr=uint8
  OMAPve_y_Prefill_requestNum : Constant  Value=0  OutDataTypeStr=uint8
  OMAPve_y_RVVACC_Vehiclespeed_request_typeNum3 : Constant  Value=0  OutDataTypeStr=uint8
  OMAPve_y_State_of_the_functionFARC_detNum : Constant  Value=0  OutDataTypeStr=uint8
  OMAPve_y_TARGET_POSITIONNum3 : Constant  Value=6  OutDataTypeStr=uint8
  OMAPve_y_TJA_status_iconNum3 : Constant  Value=0  OutDataTypeStr=uint8
  OMAPve_y_TSR_Vision_Only_Sign_TypeNum3 : Constant  Value=0  OutDataTypeStr=uint8
  OMAPve_y_stAcvTqWhlPTPotReqNum : Constant  Value=0  OutDataTypeStr=uint8
  LKA_EMS : Outport
  LKA_ESC : Outport  Port=2
  LKA_EPS : Outport  Port=3
  LKA_IC : Outport  Port=4
  LKA_Input : Outport  Port=5
  wires:
  Bus Selector/1 -> Data Type Conversion39/1  "<FDMMve_d_LkaFcnConf_convert>"
  Bus Selector9/11 -> Data Type Conversion38/1  "<LKASve_y_LKA_Action_Indication_convert>"
  Bus Selector9/4 -> Data Type Conversion31/1  "<LKASve_y_EPS_LKA_Control_convert>"
  OMAPve_y_TSR_Vision_Only_Sign_TypeNum3/1 -> Bus Creator1/8  "OMAPve_y_TSR_Vision_Only_Sign_Type_2"
  Bus Selector9/5 -> Data Type Conversion32/1  "<LKASve_y_Hands_Off_Warning_convert>"
  Data Type Conversion39/1 -> Bus Creator1/32  "OMAPve_y_LKA_Switch_State_2"
  Data Type Conversion34/1 -> Bus Creator1/27  "OMAPve_y_Vehicle_Lane_Display_2"
  Bus Selector9/10 -> Data Type Conversion37/1  "<LKASve_y_LKA_Status_Display_convert>"
  Bus Creator12/1 -> LKA_EPS/1  "LKA_EPS"
  Bus Selector9/6 -> Data Type Conversion33/1  "<LKASve_y_HMI_Popup_Status_convert>"
  Data Type Conversion32/1 -> Bus Creator1/25  "OMAPve_y_Hands_off_warning_2"
  Input_FDMM/1 -> Bus Selector/1
  Constant22/1 -> Bus Creator1/30  "OMAPve_y_LKA_Mode_from_Camera_2"
  Constant21/1 -> Bus Creator12/1  "OMAPve_y_Power_steering_power_cut3F2_2"
  OMAPve_y_TJA_status_iconNum3/1 -> Bus Creator1/36  "OMAPve_y_TJA_status_icon_2"
  Data Type Conversion29/1 -> Bus Creator12/3  "OMAPve_g_Coefficient_toregulate_EPS_2"
  Input_LKAS/1 -> LKA_Input/1, Bus Selector9/1
  OMAPve_y_ACC_DesiredHeadway_DisplayNum3/1 -> Bus Creator1/9  "OMAPve_y_ACC_DesiredHeadway_Display_2"
  OMAPve_y_ACC_Pop_Up_MessageNum3/1 -> Bus Creator1/15  "OMAPve_y_ACC_Pop_Up_Message_2"
  OMAPve_y_ACC_Vehicle_Icon_DisplayNum3/1 -> Bus Creator1/13  "OMAPve_y_ACC_Vehicle_Icon_Display_2"
  Bus Selector9/8 -> Data Type Conversion35/1  "<LKASve_y_LDW_Flag_convert>"
  OMAPve_y_ICA_HMI_Txt_DispNum3/1 -> Bus Creator1/35  "OMAPve_y_ICA_HMI_Txt_Disp_2"
  OMAPve_y_TARGET_POSITIONNum3/1 -> Bus Creator1/22  "OMAPve_y_TARGET_POSITION_2"
  Data Type Conversion37/1 -> Bus Creator1/31  "OMAPve_y_LKA_Status_Display_2"
  OMAPve_y_RVVACC_Vehiclespeed_request_typeNum3/1 -> Bus Creator1/14  "OMAPve_y_RVVACC_Vehiclespeed_request_type_2"
  Data Type Conversion36/1 -> Bus Creator1/29  "OMAPve_y_LDW_Status_Display_2"
  Data Type Conversion38/1 -> Bus Creator1/33  "OMAPve_y_LKA_action_indication_2"
  OMAPve_y_AEB_Switch_StatusNum1/1 -> Bus Creator1/18  "OMAPve_y_AEB_Switch_Status_2"
  Bus Selector9/2 -> Data Type Conversion29/1  "<LKASve_g_EPS_Factor_Control_convert>"
  Data Type Conversion33/1 -> Bus Creator1/26  "OMAPve_y_HMI_Popup_Status_2"
  OMAPve_y_AEB_Fault_StatusNum1/1 -> Bus Creator1/17  "OMAPve_y_AEB_Fault_Status_2"
  OMAPve_y_ACC_Set_Speed_DisplayNum3/1 -> Bus Creator1/12  "OMAPve_y_ACC_Set_Speed_Display_2"
  Bus Selector9/1 -> Data Type Conversion28/1  "<LKASve_y_EPS_State_Control_convert>"
  OMAPve_y_ACC_HMI_TgtDisp_FlagNum3/1 -> Bus Creator1/21  "OMAPve_y_ACC_HMI_TgtDisp_Flag_2"
  Data Type Conversion28/1 -> Bus Creator12/2  "OMAPve_y_General_state_of_LKA_function3F2_2"
  Bus Selector9/7 -> Data Type Conversion34/1  "<LKASve_y_Vehicle_Lane_Display_convert>"
  Data Type Conversion31/1 -> Bus Creator12/5  "OMAPve_y_Permit_to_know_if_LKA_or_LPA3F2_2"
  OMAPve_y_ACC_DesiredHeadway_Icon_BasicNum3/1 -> Bus Creator1/10  "OMAPve_y_ACC_DesiredHeadway_Icon_Basic_2"
  Data Type Conversion35/1 -> Bus Creator1/28  "OMAPve_y_LDW_Flag_2"
  OMAPve_y_ACC_Desired_Set_SpeedNum3/1 -> Bus Creator1/11  "OMAPve_y_ACC_Desired_Set_Speed_2"
  Data Type Conversion30/1 -> Bus Creator12/4  "OMAPve_g_Column_angle_setpoint3F2_2"
  Bus Selector9/3 -> Data Type Conversion30/1  "<LKASve_g_LKA_SWA_Control_convert>"
  Bus Selector9/9 -> Data Type Conversion36/1  "<LKASve_y_LDW_Status_Display_convert>"
  OMAPve_y_AEB_tipsNum1/1 -> Bus Creator1/19  "OMAPve_y_AEB_tips_2"
  OMAPve_y_AEB_Alert_ReqNum1/1 -> Bus Creator1/16  "OMAPve_y_AEB_Alert_Req_2"
  OMAPve_g_TminUp_or_downGearNum/1 -> Bus Creator/5  "OMAPve_g_TminUp_or_downGear_1"
  Bus Creator/1 -> LKA_EMS/1  "LKA_EMS"
  OMAPve_g_PotACCTqReqNum/1 -> Bus Creator/2  "OMAPve_g_PotACCTqReq_1"
  OMAPve_y_Powertrain_torquewheel_requestNum/1 -> Bus Creator/4  "OMAPve_y_Powertrain_torquewheel_request_1"
  OMAPve_g_ACCTqReqNum/1 -> Bus Creator/3  "OMAPve_g_ACCTqReq_1"
  OMAPve_y_ACC_Engine_Start_RequestNum/1 -> Bus Creator/1  "OMAPve_y_ACC_Engine_Start_Request_1"
  OMAPve_y_Function_Acc_statusNum/1 -> Bus Creator/7  "OMAPve_y_Function_Acc_status_1"
  OMAPve_y_stAcvTqWhlPTPotReqNum/1 -> Bus Creator/6  "OMAPve_y_stAcvTqWhlPTPotReq_1"
  OMAPve_y_MDD_deceleration_typeNum/1 -> Bus Creator5/10  "OMAPve_y_MDD_deceleration_type_1"
  OMAPve_y_MDD_Decelerationcontrol_requestNum/1 -> Bus Creator5/9  "OMAPve_y_MDD_Decelerationcontrol_request_1"
  OMAPve_y_Decel_RequestNum/1 -> Bus Creator5/11  "OMAPve_y_Decel_Request_1"
  OMAPve_y_Prefill_requestNum/1 -> Bus Creator5/4  "OMAPve_y_Prefill_request_1"
  OMAPve_g_Deceleration_setpoint_deviceNum/1 -> Bus Creator5/8  "OMAPve_g_Deceleration_setpoint_device_1"
  OMAPve_y_AEB_StatusNum/1 -> Bus Creator5/3  "OMAPve_y_AEB_Status_1"
  OMAPve_y_AEB_Braking_progressNum/1 -> Bus Creator5/12  "OMAPve_y_AEB_Braking_progress_1"
  OMAPve_y_FCW_StatusNum/1 -> Bus Creator5/1  "OMAPve_y_FCW_Status_1"
  OMAPve_y_State_of_the_functionFARC_detNum/1 -> Bus Creator5/2  "OMAPve_y_State_of_the_functionFARC_det_1"
  OMAPve_y_Haptic_AlarmNum/1 -> Bus Creator5/5  "OMAPve_y_Haptic_Alarm_1"
  Bus Creator5/1 -> LKA_ESC/1  "LKA_ESC"
  OMAPve_y_ADAS_ELKStsNum1/1 -> Bus Creator1/34  "OMAPve_y_ADAS_ELKSts_2"
  OMAPve_y_ADAS_ESCHoldReqNum/1 -> Bus Creator5/7  "OMAPve_y_ADAS_ESCHoldReq"
  OMAPve_y_ADAS_ESCDriveOffNum/1 -> Bus Creator5/6  "OMAPve_y_ADAS_ESCDriveOff"
  OMAPve_y_ADAS_ACCRequestEPBNum/1 -> Bus Creator5/13  "OMAPve_y_ADAS_ACCRequestEPB"
  OMAPve_y_ADAS_JAFaultSt_2/1 -> Bus Creator1/20  "OMAPve_y_ADAS_JAFaultSt_2"
  OMAPve_y_ADAS_ISLCState1/1 -> Bus Creator1/23  "OMAPve_y_ADAS_ISLCState_2"
  OMAPve_y_ADAS_ISLCDriverRemind1/1 -> Bus Creator1/24  "OMAPve_y_ADAS_ISLCDriverRemind_2"
  OMAPve_y_ADAS_LightControlValid/1 -> Bus Creator1/6  "OMAPve_y_ADAS_LightControlValid_2"
  OMAPve_y_ADAS_HWAActionSts/1 -> Bus Creator1/4  "OMAPve_y_ADAS_HWAActionSts_2"
  OMAPve_y_ADAS_HWATurnOnIndicator/1 -> Bus Creator1/3  "OMAPve_y_ADAS_HWATurnOnIndicator_2"
  OMAPve_y_ADAS_HWAMode/1 -> Bus Creator1/7  "OMAPve_y_ADAS_HWAMode_2"
  OMAPve_y_ADAS_TurnLightsCommand1/1 -> Bus Creator1/5  "OMAPve_y_ADAS_TurnLightsCommand_2"
  Constant1/1 -> Bus Creator12/7  "OMAPve_g_ADAS_ESATorqueReq_2"
  Constant/1 -> Bus Creator12/6  "OMAPve_y_ADAS_ESAState_2"
  Constant2/1 -> Bus Creator12/8  "OMAPve_y_ADAS_ESARequest_2"
  Constant3/1 -> Bus Creator1/2  "OMAPve_y_ADAS_ESAFaultSt_2"
  Constant5/1 -> Bus Creator1/1  "OMAPve_y_ADAS_ELKPopupMessage_2"
  Bus Creator1/1 -> LKA_IC/1  "LKA_IC"

== system MIL4L3_SW6_V1_20220211/CarMaker/VehicleControl/OMAP/OMAP1/Runnable_OMAP_10ms_sys/OMAP_Module/OTHER_Default_Arbitration ==
  Bus Creator27 : BusCreator  Inputs=5
  Data Type Conversion72 : DataTypeConversion  OutDataTypeStr=uint8
  Delay : Delay
  NOT : Logic  Operator=NOT  IconShape=distinctive  AllPortsSameDT=off  OutDataTypeStr=boolean
  OMAPve_y_ABS_ESP_power_cut_request2Num1 : Constant  Value=0  OutDataTypeStr=uint8
  OMAPve_y_ASR_connection_dis_demand2Num1 : Constant  Value=0  OutDataTypeStr=uint8
  OMAPve_y_ECU_operating_phaseNum1 : Constant  Value=9  OutDataTypeStr=uint8
  OMAPve_y_Radar_StateNum1 : Constant  Value=2  OutDataTypeStr=uint8
  Arbitration : Outport
  wires:
  Bus Creator27/1 -> Arbitration/1  "Arbitration"
  Data Type Conversion72/1 -> Bus Creator27/3  "OMAPve_y_TYPE_RAPPORT_2"
  Delay/1 -> NOT/1
  OMAPve_y_ASR_connection_dis_demand2Num1/1 -> Bus Creator27/2  "OMAPve_y_ASR_connection_dis_demand2_2"
  OMAPve_y_ABS_ESP_power_cut_request2Num1/1 -> Bus Creator27/1  "OMAPve_y_ABS_ESP_power_cut_request2_2"
  OMAPve_y_ECU_operating_phaseNum1/1 -> Bus Creator27/4  "OMAPve_y_ECU_operating_phase_2"
  OMAPve_y_Radar_StateNum1/1 -> Bus Creator27/5  "OMAPve_y_Radar_State_2"
  NOT/1 -> Delay/1, Data Type Conversion72/1

== system MIL4L3_SW6_V1_20220211/CarMaker/VehicleControl/OMAP/OMAP1/Runnable_OMAP_10ms_sys/OMAP_Module/Subsystem1 ==
  In1 : Inport
  Constant : Constant  Value=6  OutDataTypeStr=uint8
  Constant1 : Constant  Value=0  OutDataTypeStr=uint8
  Index Vector1 : MultiPortSwitch  DataPortOrder=Specify indices  Inputs=11  DataPortIndices={6,0}  DiagnosticForDefault=None  OutDataTypeStr=uint8
  Out1 : Outport
  wires:
  Index Vector1/1 -> Out1/1
  In1/1 -> Index Vector1/1
  Constant/1 -> Index Vector1/2
  Constant1/1 -> Index Vector1/3
